simulink model "array_task"  (R2021a)
settings: Solver=FixedStepDiscrete  StartTime=0.0  StopTime=10.0  RelTol=1e-3  EnableMultiTasking=on
settings Model: Creator=omar  LastModifiedBy=omar
settings DataIOCC: ReturnWorkspaceOutputs=off
settings OptimizationCC: DefaultParameterBehavior=Inlined  InlineInvariantSignals=on  EnableMemcpy=off  LifeSpan=1  EfficientTunableParamExpr=on
settings DebuggingCC: UnderspecifiedInitializationDetection=Classic  MergeDetectMultiDrivingBlocksExec=none  SFMachineParentedDataDiag=warning  ArithmeticOperatorsInVariantConditions=warning
settings ModelReferenceCC: PropagateSignalLabelsOutOfModel=off
settings SFSimCC: MATLABDynamicMemAlloc=off  CustomCodeUndefinedFunction=UseInterfaceOnly
settings RTWCC: SystemTargetFile=ert.tlc  GenCodeOnly=on  TemplateMakefile=ert_default_tmf  GenerateReport=on  IncludeHyperlinkInReport=on  LaunchReport=on  GenerateTraceInfo=on  GenerateTraceReport=on  GenerateTraceReportSl=on  GenerateTraceReportSf=on  GenerateTraceReportEml=on
settings CodeAppCC: ForceParamTrailComments=on  IgnoreCustomStorageClasses=off  OperatorAnnotations=on  SimulinkDataObjDesc=on  SFDataObjDesc=on  MATLABFcnDesc=on  InsertBlockDesc=on  StateflowObjectComments=on  MATLABSourceComments=on
settings ERTTargetCC: MultiwordLength=2048  GenerateSampleERTMain=on  InlinedParameterPlacement=NonHierarchical  ERTCustomFileTemplate=example_file_process.tlc

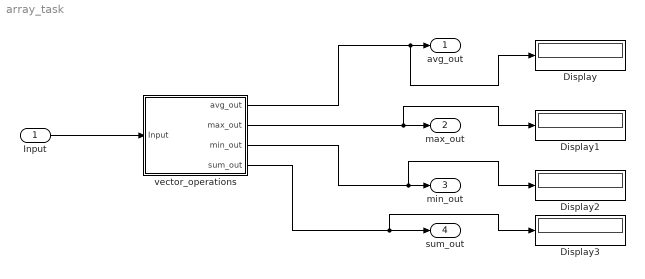
== system array_task ==
  Input : Inport
  Display{,1..3} (4 alike) : Display
  vector_operations : Subsystem
  avg_out : Outport
  max_out : Outport  Port=2
  min_out : Outport  Port=3
  sum_out : Outport  Port=4
  wires:
  vector_operations/1(avg_out) -> Display/1, avg_out/1
  vector_operations/2(max_out) -> Display1/1, max_out/1
  vector_operations/3(min_out) -> Display2/1, min_out/1
  vector_operations/4(sum_out) -> Display3/1, sum_out/1
  Input/1 -> vector_operations/1(Input)

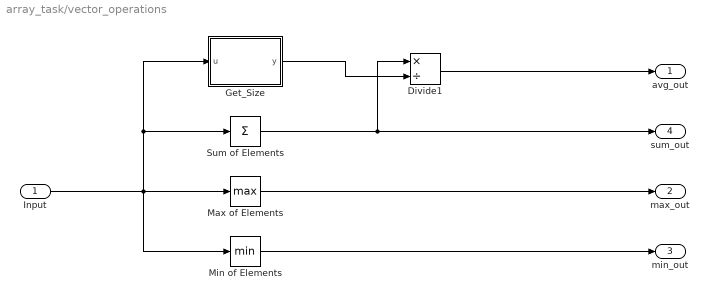
== system array_task/vector_operations ==
  Input : Inport
  Divide1 : Product  Inputs=*/  OutDataTypeStr=double
  Get_Size : MATLAB Function  TreatAsAtomicUnit=on
  Max of Elements : MinMax  Function=max
  Min of Elements : MinMax
  Sum of Elements : Sum  Inputs=+
  avg_out : Outport
  max_out : Outport  Port=2
  min_out : Outport  Port=3
  sum_out : Outport  Port=4
  wires:
  Divide1/1 -> avg_out/1
  Input/1 -> Get_Size/1(u), Sum of Elements/1, Max of Elements/1, Min of Elements/1
  Max of Elements/1 -> max_out/1
  Sum of Elements/1 -> Divide1/1, sum_out/1
  Min of Elements/1 -> min_out/1
  Get_Size/1(y) -> Divide1/2

== matlab function array_task/vector_operations/Get_Size ==
  data: u input; y output
function y = GetSize(u)
y = length(u);
